simulink model "LIPM_Dynamicsy_3Mass"  (R2020a)
settings: Solver=ode3  StartTime=0.0  StopTime=0.65  FixedStep=t_sample  RelTol=1e-3  EnableMultiTasking=on
values from neighbouring files (symbols this model uses):
  n = length(Step)-1    [3mass1mass.m]    (also in Ctrl_body_eng.m; ONEmassONEmass.m; THREEmassONEmass.m; THREEmassTHREEmass.m)
  omega = 3.5    [3mass1mass.m]    (also in Ctrl_body_eng.m = sqrt(g/delta_z_vrp); ONEmassONEmass.m; THREEmassONEmass.m; THREEmassTHREEmass.m)
  V0_3Mass = V0_3Mass + t_sample*(omega^2*(x0_3Mass-zmp_pend(ini(n+1)-1+q,1:2)')+[0;-F/m])    [3mass1mass.m]    (also in Ctrl_body_eng.m = omega*(term1_3Mass-term2_3Mass); ONEmassONEmass.m = V0_3Mass + t_sample*(omega^2*(x0_3Mass-(u0+[PcZMP_x(q,n+1);P; THREEmassONEmass.m = V0_3Mass + t_sample*(omega^2*(x0_3Mass-(zmp_pend(ini(n+1)-1+; THREEmassTHREEmass.m = V0_3Mass + t_sample*(omega^2*(x0_3Mass-(zmp_pend(ini(n+1)-1+)
  x0_3Mass = [xi_ini(1,1) xi_ini(1,2)]'    [3mass1mass.m]    (also in Ctrl_body_eng.m = [CoM_x_3Mass(2) CoM_y_3Mass(2)]'; ONEmassONEmass.m; THREEmassONEmass.m; THREEmassTHREEmass.m)
  zmp_pend = [time; (m/mpend)*[u0_x(2); u0_y(2)] - (mfeet/mpend)*zmp_feet(2:3)]    [Ctrl_body_eng.m]
settings Model: Creator=Fateme  LastModifiedBy=zakaria
settings DataIOCC: LimitDataPoints=on  SaveFormat=Array  ReturnWorkspaceOutputs=off
settings OptimizationCC: LifeSpan=inf
settings DebuggingCC: SolverPrmCheckMsg=warning  SFUnexpectedBacktrackingDiag=warning  SFNoUnconditionalDefaultTransitionDiag=warning  SFExecutionAtInitializationDiag=none  ArithmeticOperatorsInVariantConditions=warning
settings HardwareCC: ProdBitPerPointer=32  ProdBitPerSizeT=32  ProdBitPerPtrDiffT=32  ProdLargestAtomicFloat=None  ProdIntDivRoundTo=Undefined  ProdEndianess=Unspecified  ProdWordSize=32  ProdHWDeviceType=32-bit Generic
settings ModelReferenceCC: PropagateSignalLabelsOutOfModel=off
settings SFSimCC: SimUseLocalCustomCode=off  CustomCodeUndefinedFunction=UseInterfaceOnly
settings RTWCC: RTWUseLocalCustomCode=off
settings CodeAppCC: StateflowObjectComments=on
settings GRTTargetCC: TargetLangStandard=C89/C90 (ANSI)
settings ConfigComp: CovMetricSettings=dw  CovHtmlReporting=on  CovSaveCumulativeToWorkspaceVar=on  CovSaveSingleToWorkspaceVar=on  CovExternalEMLEnable=off  CovSFcnEnable=off

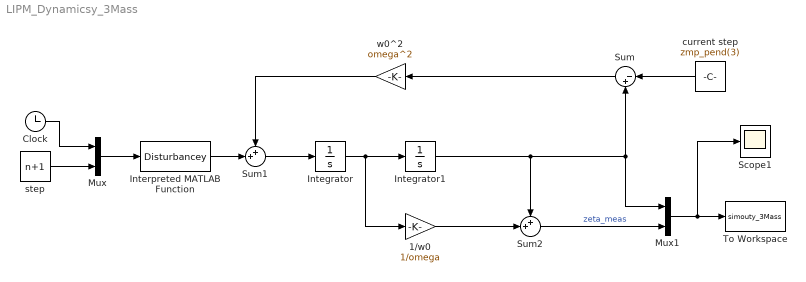
== system LIPM_Dynamicsy_3Mass ==
  1/w0 : Gain  Gain=1/omega
  Clock : Clock
  Integrator : Integrator  InitialCondition=V0_3Mass(2)
  Integrator1 : Integrator  InitialCondition=x0_3Mass(2)
  Interpreted MATLAB Function : MATLABFcn  MATLABFcn=Disturbancey
  Mux : Mux  Inputs=2
  Mux1 : Mux  Inputs=2
  Scope1 : Scope
  Sum : Sum  Inputs=|-+
  Sum1 : Sum  Inputs=++|
  Sum2 : Sum  Inputs=++|
  To Workspace : ToWorkspace  VariableName=simouty_3Mass  SampleTime=-1
  current step : Constant  Value=zmp_pend(3)
  step : Constant  Value=n+1
  w0^2 : Gain  Gain=omega^2
  wires:
  Integrator/1 -> 1/w0/1, Integrator1/1
  Integrator1/1 -> Sum2/1, Mux1/1, Sum/2
  current step/1 -> Sum/1
  Sum/1 -> w0^2/1
  w0^2/1 -> Sum1/1
  Sum1/1 -> Integrator/1
  Mux/1 -> Interpreted MATLAB Function/1
  Clock/1 -> Mux/1
  step/1 -> Mux/2
  Mux1/1 -> Scope1/1, To Workspace/1
  Sum2/1 -> Mux1/2  "zeta_meas"
  1/w0/1 -> Sum2/2
  Interpreted MATLAB Function/1 -> Sum1/2
